simulink model "y005"  (R2019b)
settings: Solver=ode23tb  StartTime=0.0  StopTime=1  MaxStep=0.00001  RelTol=1e-3
values from neighbouring files (symbols this model uses):
  fN = 50    [parameter.m]
  J = 0.1284    [parameter.m]
  Llr = Lr - Lm    (= 0.006)    [parameter.m]
  Lls = Ls - Lm    (= 0.0102)    [parameter.m]
  np = 2    [parameter.m]
  PN = 3000    [parameter.m]
  Rr = 2.685    [parameter.m]
  Rs = 1.85    [parameter.m]
  TN = PN/(2*pi*nN/60)    (= 20.4627783975)    [parameter.m]
  UN = 380    [parameter.m]
undefined symbols (not defined in the file or in its folder): i
libraries: simulink x9, powerlib x9
Description:
  | SVPWM调制
settings Model: Creator=Inspiron  LastModifiedBy=Inspiron
settings SolverCC: ZeroCrossAlgorithm=Adaptive
settings DebuggingCC: IgnoredZcDiagnostic=none

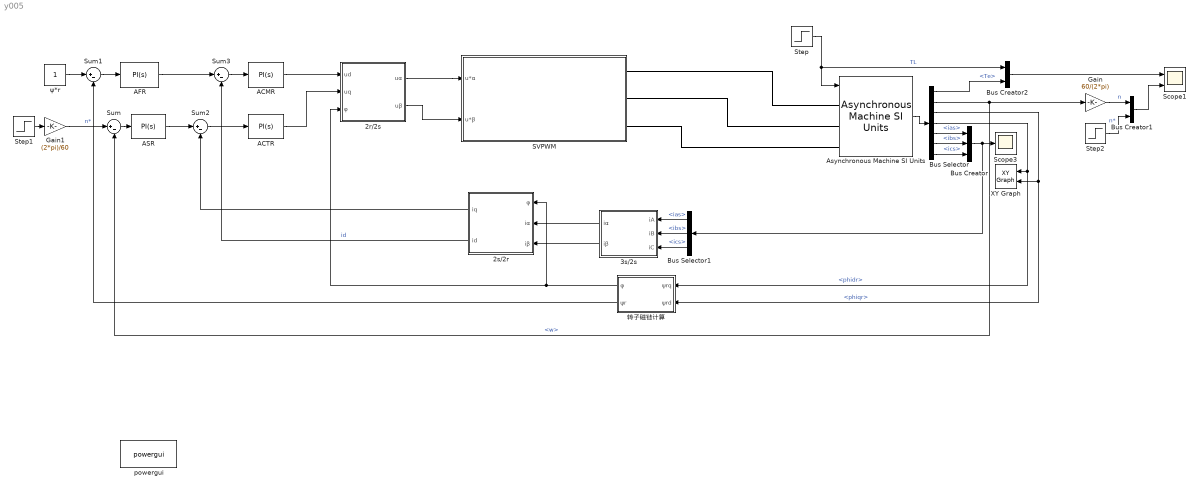
== system y005 ==
  2r/2s : Subsystem
  2s/2r : Subsystem
  3s/2s : Subsystem
  ACMR : simulink/Continuous/PID Controller  Controller=PI  Form=Parallel  TimeDomain=Continuous-time  SampleTime=-1  IntegratorMethod=Forward Euler  FilterMethod=Forward Euler  ControllerParametersSource=internal  P=30  I=2  D=0  UseFilter=on  N=100  TunerSelectOption=Transfer Function Based (PID Tuner App)  InitialConditionSource=internal  InitialConditionForIntegrator=0  InitialConditionForFilter=0  DifferentiatorICPrevScaledInput=0  ExternalReset=none  TrackingMode=off  Kt=1  LimitOutput=on  UpperSaturationLimit=500  LowerSaturationLimit=-500  LinearizeAsGain=on  AntiWindupMode=none  Kb=1  POutMin=[]  POutMax=[]  IOutMin=[]  IOutMax=[]  DOutMin=[]  DOutMax=[]  NOutMin=[]  NOutMax=[]  SumOutMin=[]  SumOutMax=[]  SaturationOutMin=[]  SaturationOutMax=[]  PParamMin=[]  PParamMax=[]  IParamMin=[]  IParamMax=[]  DParamMin=[]  DParamMax=[]  NParamMin=[]  NParamMax=[]  KbParamMin=[]  KbParamMax=[]  KtParamMin=[]  KtParamMax=[]  KbOutMin=[]  KbOutMax=[]  KtOutMin=[]  KtOutMax=[]  IntegratorOutMin=[]  IntegratorOutMax=[]  FilterOutMin=[]  FilterOutMax=[]  SumI1OutMin=[]  SumI1OutMax=[]  SumI2OutMin=[]  SumI2OutMax=[]  SumI3OutMin=[]  SumI3OutMax=[]  SumI4OutMin=[]  SumI4OutMax=[]  SumDOutMin=[]  SumDOutMax=[]  DifferentiatorOutMin=[]  DifferentiatorOutMax=[]  FilterDiffOutCoefMin=[]  FilterDiffOutCoefMax=[]  ReciprocalOutMin=[]  ReciprocalOutMax=[]  SumDenOutMin=[]  SumDenOutMax=[]  SumNumOutMin=[]  SumNumOutMax=[]  DivideOutMin=[]  DivideOutMax=[]  IntegratorContinuousStateAttributes=''  IntegratorStateMustResolveToSignalObject=off  IntegratorRTWStateStorageClass=Auto  FilterContinuousStateAttributes=''  FilterStateMustResolveToSignalObject=off  FilterRTWStateStorageClass=Auto  ParallelPVariant=InternalParameters  IdealPVariant=Disabled  IVariant=InternalParameters  DVariant=Disabled  IntegratorVariant=Continuous  SatVariant=Enabled  AWVariant=Passthrough  PCopyVariant=Disabled  TRVariant=Disabled  FdbkBlocksVariant=Forward  IdealPFdbkVariant=Disabled  SatFdbkVariant=Disabled  DerivativeFilterVariant=Disabled  NVariant=Disabled  NCopyVariant=Disabled_SignalSpec  FilterICVariant=Disabled  IntegratorICVariant=InternalICs  ExternalResetVariant=Disabled  TRSumVariant=Passthrough  SumFdbkVariant=Disabled  SumVariant=Sum_PI
  ACTR : simulink/Continuous/PID Controller  Controller=PI  Form=Parallel  TimeDomain=Continuous-time  SampleTime=-1  IntegratorMethod=Forward Euler  FilterMethod=Forward Euler  ControllerParametersSource=internal  P=50  I=10  D=0  UseFilter=on  N=100  TunerSelectOption=Transfer Function Based (PID Tuner App)  InitialConditionSource=internal  InitialConditionForIntegrator=0  InitialConditionForFilter=0  DifferentiatorICPrevScaledInput=0  ExternalReset=none  TrackingMode=off  Kt=1  LimitOutput=on  UpperSaturationLimit=500  LowerSaturationLimit=-500  LinearizeAsGain=on  AntiWindupMode=none  Kb=1  POutMin=[]  POutMax=[]  IOutMin=[]  IOutMax=[]  DOutMin=[]  DOutMax=[]  NOutMin=[]  NOutMax=[]  SumOutMin=[]  SumOutMax=[]  SaturationOutMin=[]  SaturationOutMax=[]  PParamMin=[]  PParamMax=[]  IParamMin=[]  IParamMax=[]  DParamMin=[]  DParamMax=[]  NParamMin=[]  NParamMax=[]  KbParamMin=[]  KbParamMax=[]  KtParamMin=[]  KtParamMax=[]  KbOutMin=[]  KbOutMax=[]  KtOutMin=[]  KtOutMax=[]  IntegratorOutMin=[]  IntegratorOutMax=[]  FilterOutMin=[]  FilterOutMax=[]  SumI1OutMin=[]  SumI1OutMax=[]  SumI2OutMin=[]  SumI2OutMax=[]  SumI3OutMin=[]  SumI3OutMax=[]  SumI4OutMin=[]  SumI4OutMax=[]  SumDOutMin=[]  SumDOutMax=[]  DifferentiatorOutMin=[]  DifferentiatorOutMax=[]  FilterDiffOutCoefMin=[]  FilterDiffOutCoefMax=[]  ReciprocalOutMin=[]  ReciprocalOutMax=[]  SumDenOutMin=[]  SumDenOutMax=[]  SumNumOutMin=[]  SumNumOutMax=[]  DivideOutMin=[]  DivideOutMax=[]  IntegratorContinuousStateAttributes=''  IntegratorStateMustResolveToSignalObject=off  IntegratorRTWStateStorageClass=Auto  FilterContinuousStateAttributes=''  FilterStateMustResolveToSignalObject=off  FilterRTWStateStorageClass=Auto  ParallelPVariant=InternalParameters  IdealPVariant=Disabled  IVariant=InternalParameters  DVariant=Disabled  IntegratorVariant=Continuous  SatVariant=Enabled  AWVariant=Passthrough  PCopyVariant=Disabled  TRVariant=Disabled  FdbkBlocksVariant=Forward  IdealPFdbkVariant=Disabled  SatFdbkVariant=Disabled  DerivativeFilterVariant=Disabled  NVariant=Disabled  NCopyVariant=Disabled_SignalSpec  FilterICVariant=Disabled  IntegratorICVariant=InternalICs  ExternalResetVariant=Disabled  TRSumVariant=Passthrough  SumFdbkVariant=Disabled  SumVariant=Sum_PI
  AFR : simulink/Continuous/PID Controller  Controller=PI  Form=Parallel  TimeDomain=Continuous-time  SampleTime=-1  IntegratorMethod=Forward Euler  FilterMethod=Forward Euler  ControllerParametersSource=internal  P=80  I=20  D=0  UseFilter=on  N=100  TunerSelectOption=Transfer Function Based (PID Tuner App)  InitialConditionSource=internal  InitialConditionForIntegrator=0  InitialConditionForFilter=0  DifferentiatorICPrevScaledInput=0  ExternalReset=none  TrackingMode=off  Kt=1  LimitOutput=on  UpperSaturationLimit=40  LowerSaturationLimit=-40  LinearizeAsGain=on  AntiWindupMode=none  Kb=1  POutMin=[]  POutMax=[]  IOutMin=[]  IOutMax=[]  DOutMin=[]  DOutMax=[]  NOutMin=[]  NOutMax=[]  SumOutMin=[]  SumOutMax=[]  SaturationOutMin=[]  SaturationOutMax=[]  PParamMin=[]  PParamMax=[]  IParamMin=[]  IParamMax=[]  DParamMin=[]  DParamMax=[]  NParamMin=[]  NParamMax=[]  KbParamMin=[]  KbParamMax=[]  KtParamMin=[]  KtParamMax=[]  KbOutMin=[]  KbOutMax=[]  KtOutMin=[]  KtOutMax=[]  IntegratorOutMin=[]  IntegratorOutMax=[]  FilterOutMin=[]  FilterOutMax=[]  SumI1OutMin=[]  SumI1OutMax=[]  SumI2OutMin=[]  SumI2OutMax=[]  SumI3OutMin=[]  SumI3OutMax=[]  SumI4OutMin=[]  SumI4OutMax=[]  SumDOutMin=[]  SumDOutMax=[]  DifferentiatorOutMin=[]  DifferentiatorOutMax=[]  FilterDiffOutCoefMin=[]  FilterDiffOutCoefMax=[]  ReciprocalOutMin=[]  ReciprocalOutMax=[]  SumDenOutMin=[]  SumDenOutMax=[]  SumNumOutMin=[]  SumNumOutMax=[]  DivideOutMin=[]  DivideOutMax=[]  IntegratorContinuousStateAttributes=''  IntegratorStateMustResolveToSignalObject=off  IntegratorRTWStateStorageClass=Auto  FilterContinuousStateAttributes=''  FilterStateMustResolveToSignalObject=off  FilterRTWStateStorageClass=Auto  ParallelPVariant=InternalParameters  IdealPVariant=Disabled  IVariant=InternalParameters  DVariant=Disabled  IntegratorVariant=Continuous  SatVariant=Enabled  AWVariant=Passthrough  PCopyVariant=Disabled  TRVariant=Disabled  FdbkBlocksVariant=Forward  IdealPFdbkVariant=Disabled  SatFdbkVariant=Disabled  DerivativeFilterVariant=Disabled  NVariant=Disabled  NCopyVariant=Disabled_SignalSpec  FilterICVariant=Disabled  IntegratorICVariant=InternalICs  ExternalResetVariant=Disabled  TRSumVariant=Passthrough  SumFdbkVariant=Disabled  SumVariant=Sum_PI
  ASR : simulink/Continuous/PID Controller  Controller=PI  Form=Parallel  TimeDomain=Continuous-time  SampleTime=-1  IntegratorMethod=Forward Euler  FilterMethod=Forward Euler  ControllerParametersSource=internal  P=15  I=5  D=0  UseFilter=on  N=100  TunerSelectOption=Transfer Function Based (PID Tuner App)  InitialConditionSource=internal  InitialConditionForIntegrator=0  InitialConditionForFilter=0  DifferentiatorICPrevScaledInput=0  ExternalReset=none  TrackingMode=off  Kt=1  LimitOutput=on  UpperSaturationLimit=40  LowerSaturationLimit=-40  LinearizeAsGain=on  AntiWindupMode=none  Kb=1  POutMin=[]  POutMax=[]  IOutMin=[]  IOutMax=[]  DOutMin=[]  DOutMax=[]  NOutMin=[]  NOutMax=[]  SumOutMin=[]  SumOutMax=[]  SaturationOutMin=[]  SaturationOutMax=[]  PParamMin=[]  PParamMax=[]  IParamMin=[]  IParamMax=[]  DParamMin=[]  DParamMax=[]  NParamMin=[]  NParamMax=[]  KbParamMin=[]  KbParamMax=[]  KtParamMin=[]  KtParamMax=[]  KbOutMin=[]  KbOutMax=[]  KtOutMin=[]  KtOutMax=[]  IntegratorOutMin=[]  IntegratorOutMax=[]  FilterOutMin=[]  FilterOutMax=[]  SumI1OutMin=[]  SumI1OutMax=[]  SumI2OutMin=[]  SumI2OutMax=[]  SumI3OutMin=[]  SumI3OutMax=[]  SumI4OutMin=[]  SumI4OutMax=[]  SumDOutMin=[]  SumDOutMax=[]  DifferentiatorOutMin=[]  DifferentiatorOutMax=[]  FilterDiffOutCoefMin=[]  FilterDiffOutCoefMax=[]  ReciprocalOutMin=[]  ReciprocalOutMax=[]  SumDenOutMin=[]  SumDenOutMax=[]  SumNumOutMin=[]  SumNumOutMax=[]  DivideOutMin=[]  DivideOutMax=[]  IntegratorContinuousStateAttributes=''  IntegratorStateMustResolveToSignalObject=off  IntegratorRTWStateStorageClass=Auto  FilterContinuousStateAttributes=''  FilterStateMustResolveToSignalObject=off  FilterRTWStateStorageClass=Auto  ParallelPVariant=InternalParameters  IdealPVariant=Disabled  IVariant=InternalParameters  DVariant=Disabled  IntegratorVariant=Continuous  SatVariant=Enabled  AWVariant=Passthrough  PCopyVariant=Disabled  TRVariant=Disabled  FdbkBlocksVariant=Forward  IdealPFdbkVariant=Disabled  SatFdbkVariant=Disabled  DerivativeFilterVariant=Disabled  NVariant=Disabled  NCopyVariant=Disabled_SignalSpec  FilterICVariant=Disabled  IntegratorICVariant=InternalICs  ExternalResetVariant=Disabled  TRSumVariant=Passthrough  SumFdbkVariant=Disabled  SumVariant=Sum_PI
  Asynchronous Machine SI Units : powerlib/Machines/Asynchronous Machine SI Units  RotorType=Squirrel-cage  PresetModel=No  MechanicalLoad=Torque Tm  ShowDetailedParameters=on  ReferenceFrame=Stationary  Units=SI  MeasurementBus=on  NominalParameters=[PN UN fN]  Stator=[Rs Lls]  Rotor=[Rr Llr]  Cage1=[0.4155 0.002066]  Cage2=[0.4168 0.0003495]  Lm=Lm  Mechanical=[J 0 np]  PolePairs=2  InitialConditions=[1 0 0 0 0 0 0 0]  SimulateSaturation=off  Saturation=[14.03593122, 27.81365428, 53.79336849, 72.68890987, 97.98006896, 148.6815601, 215.7428561, 302.9841135, 428.7778367 ; 230, 322, 414, 460, 506, 552, 598, 644, 690]  LoadFlowParameters=1492000  TsPowergui=0  TsBlock=-1  IterativeModel=Trapezoidal non iterative  IterativeDiscreteModel=Trapezoidal non iterative  Pmec=1.492e+006
      settings: SourceProductName=Simscape Electrical
  Bus Creator : BusCreator  Inputs=3
  Bus Creator1 : BusCreator  Inputs=2
  Bus Creator2 : BusCreator  Inputs=2
  Bus Selector : BusSelector  OutputSignals=Te,w,phiqr,phidr,ias,ibs,ics
  Bus Selector1 : BusSelector  OutputSignals=ias,ibs,ics
  Gain : Gain  Gain=60/(2*pi)
  Gain1 : Gain  Gain=(2*pi)/60
  SVPWM : Subsystem
  Scope1 : Scope  NumInputPorts=2
  Scope3 : Scope
  Step : Step  Time=0.4  After=TN  VectorParams1D=off  ZeroCross=off
  Step1 : Step  Time=0.6  Before=1000  After=0  SampleTime=0
  Step2 : Step  Time=0.6  Before=1000  After=0  SampleTime=0
  Sum{,1..3} (4 alike) : Sum  Inputs=|+-
  XY Graph : simulink/Sinks/XY Graph  xmin=-2  xmax=2  ymin=-2  ymax=2  st=-1
  powergui : powerlib/powergui  Priority=1  SimulationMode=Discrete  SampleTime=1e-5  frequency=60  Iterations=50  frequencyindice=50  Pbase=100e6  ErrMax=1e-4  UnitsV=kV  UnitsW=MW  buscounter=0  FunctionMessages=off  echomessages=off  EnableUseOfTLC=off  CurrentSourceSwitches=off  DisableSnubberDevices=off  DisableRonSwitches=off  DisableVfSwitches=off  DisplayEquations=off  AutomaticDiscreteSolvers=off  SolverType=Tustin/Backward Euler (TBE)  Interpol=off  ExternalGateDelay=off  methode=off  Ts=100  x0status=blocks  SPID=on  SwTol=0  HookPort=off  NonlinearTolerance=1e-4  nMaxIteration=100  ContinueOnMaxIteration=off  RestoreLinks=warning  ResistiveCurrentMeasurement=off  Frange=[0:2:500]  Ylog=off  Xlog=on  ShowGrid=off  save=off  variable=ZData  structure=0  ZoomFFT=off  StartTime=0.0  cycles=1  DisplayStyle=1  fundamental=60  FreqAxis=off  MaxFrequency=1000  frequencyindicesteady=1  RmsSteady=1  display=off
      settings: SourceProductName=Simscape Electrical
  ψ*r : Constant
  转子磁链计算 : Subsystem
  wires:
  Asynchronous Machine SI Units/1 -> Bus Selector/1
  Bus Creator/1 -> Scope3/1, Bus Selector1/1
  Bus Selector/5 -> Bus Creator/1  "<ias>"
  Bus Selector/6 -> Bus Creator/2  "<ibs>"
  Bus Selector/7 -> Bus Creator/3  "<ics>"
  Bus Selector/3 -> 转子磁链计算/2(ψrd), XY Graph/2  "<phiqr>"
  Bus Selector/4 -> 转子磁链计算/1(ψrq), XY Graph/1  "<phidr>"
  Sum/1 -> ASR/1
  ψ*r/1 -> Sum1/1
  Sum1/1 -> AFR/1
  Step/1 -> Bus Creator2/1, Asynchronous Machine SI Units/1  "TL"
  Step2/1 -> Bus Creator1/2  "n*"
  Bus Selector/1 -> Bus Creator2/2  "<Te>"
  Bus Creator2/1 -> Scope1/1
  Bus Creator1/1 -> Scope1/2
  Bus Selector1/1 -> 3s/2s/1(iA)  "<ias>"
  Bus Selector1/3 -> 3s/2s/3(iC)  "<ics>"
  Bus Selector1/2 -> 3s/2s/2(iB)  "<ibs>"
  Gain/1 -> Bus Creator1/1  "n"
  Bus Selector/2 -> Gain/1, Sum/2  "<w>"
  Gain1/1 -> Sum/1  "n*"
  Step1/1 -> Gain1/1
  3s/2s/1(iα) -> 2s/2r/2(iα)
  3s/2s/2(iβ) -> 2s/2r/3(iβ)
  转子磁链计算/1(φ) -> 2s/2r/1(φ), 2r/2s/3(φ)
  转子磁链计算/2(ψr) -> Sum1/2
  ASR/1 -> Sum2/1
  2s/2r/1(iq) -> Sum2/2
  AFR/1 -> Sum3/1
  2s/2r/2(id) -> Sum3/2  "id"
  Sum3/1 -> ACMR/1
  Sum2/1 -> ACTR/1
  ACMR/1 -> 2r/2s/1(ud)
  ACTR/1 -> 2r/2s/2(uq)
  2r/2s/1(uα) -> SVPWM/1(u*α)
  2r/2s/2(uβ) -> SVPWM/2(u*β)
  connections:
  Asynchronous Machine SI Units/LConn1 -- SVPWM/RConn1
  Asynchronous Machine SI Units/LConn2 -- SVPWM/RConn2
  SVPWM/RConn3 -- Asynchronous Machine SI Units/LConn3

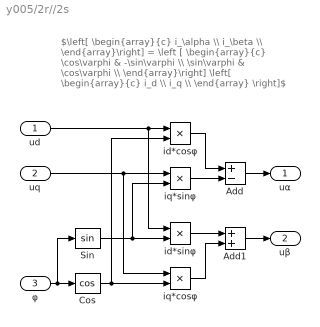
== system y005/2r//2s ==
  note: $\left[ \begin{array}{c} i_\alpha \\ i_\beta \\ \end{array}\right] = \left [ \begin{array}{c} \cos\varphi & -\sin\varphi \\ \sin\varphi & \cos\varphi \\ \end{array}\right] \left[ \begin{array}{c} i_d \\ i_q \\ \end{array} \right]$
  ud : Inport
  uq : Inport  Port=2
  φ : Inport  Port=3
  Add : Sum  Inputs=+-
  Add1 : Sum
  Cos : Trigonometry  Operator=cos
  Sin : Trigonometry
  id*cosφ : Product
  id*sinφ : Product
  iq*cosφ : Product
  iq*sinφ : Product
  uα : Outport
  uβ : Outport  Port=2
  wires:
  Cos/1 -> iq*cosφ/2, id*cosφ/2
  iq*cosφ/1 -> Add1/2
  Sin/1 -> id*sinφ/2, iq*sinφ/2
  ud/1 -> id*cosφ/1, id*sinφ/1
  id*sinφ/1 -> Add1/1
  iq*sinφ/1 -> Add/2
  uq/1 -> iq*sinφ/1, iq*cosφ/1
  φ/1 -> Sin/1, Cos/1
  Add/1 -> uα/1
  id*cosφ/1 -> Add/1
  Add1/1 -> uβ/1

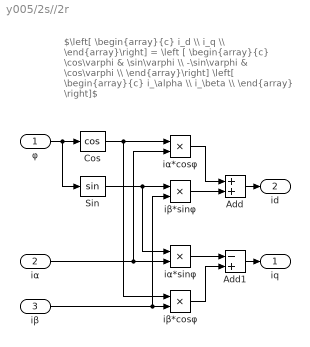
== system y005/2s//2r ==
  note: $\left[ \begin{array}{c} i_d \\ i_q \\ \end{array}\right] = \left [ \begin{array}{c} \cos\varphi & \sin\varphi \\ -\sin\varphi & \cos\varphi \\ \end{array}\right] \left[ \begin{array}{c} i_\alpha \\ i_\beta \\ \end{array} \right]$
  φ : Inport
  iα : Inport  Port=2
  iβ : Inport  Port=3
  Add : Sum
  Add1 : Sum  Inputs=-+
  Cos : Trigonometry  Operator=cos
  Sin : Trigonometry
  iα*cosφ : Product
  iα*sinφ : Product
  iβ*cosφ : Product
  iβ*sinφ : Product
  iq : Outport
  id : Outport  Port=2
  wires:
  Cos/1 -> iα*cosφ/1, iβ*cosφ/1
  iβ*cosφ/1 -> Add1/2
  Sin/1 -> iα*sinφ/1, iβ*sinφ/1
  iα/1 -> iα*sinφ/2, iα*cosφ/2
  iα*sinφ/1 -> Add1/1
  iβ*sinφ/1 -> Add/2
  iβ/1 -> iβ*sinφ/2, iβ*cosφ/2
  φ/1 -> Cos/1, Sin/1
  Add/1 -> id/1
  iα*cosφ/1 -> Add/1
  Add1/1 -> iq/1

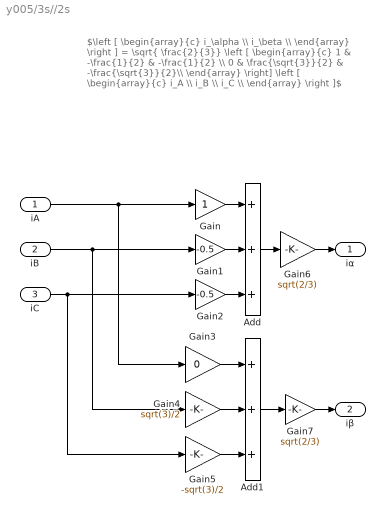
== system y005/3s//2s ==
  note: $\left [ \begin{array}{c} i_\alpha \\ i_\beta \\ \end{array} \right ] = \sqrt{ \frac{2}{3}} \left [ \begin{array}{c} 1 & -\frac{1}{2} & -\frac{1}{2} \\ 0 & \frac{\sqrt{3}}{2} & -\frac{\sqrt{3}}{2}\\ \end{array} \right] \left [ \begin{array}{c} i_A \\ i_B \\ i_C \\ \end{array} \right ]$
  iA : Inport
  iB : Inport  Port=2
  iC : Inport  Port=3
  Add : Sum  Inputs=3
  Add1 : Sum  Inputs=3
  Gain : Gain
  Gain1 : Gain  Gain=-0.5
  Gain2 : Gain  Gain=-0.5
  Gain3 : Gain  Gain=0
  Gain4 : Gain  Gain=sqrt(3)/2
  Gain5 : Gain  Gain=-sqrt(3)/2
  Gain6 : Gain  Gain=sqrt(2/3)
  Gain7 : Gain  Gain=sqrt(2/3)
  iα : Outport
  iβ : Outport  Port=2
  wires:
  Gain4/1 -> Add1/2
  Gain/1 -> Add/1
  Gain5/1 -> Add1/3
  iB/1 -> Gain4/1, Gain1/1
  Add/1 -> Gain6/1
  Gain1/1 -> Add/2
  Gain3/1 -> Add1/1
  iA/1 -> Gain3/1, Gain/1
  Gain2/1 -> Add/3
  iC/1 -> Gain5/1, Gain2/1
  Add1/1 -> Gain7/1
  Gain7/1 -> iβ/1
  Gain6/1 -> iα/1

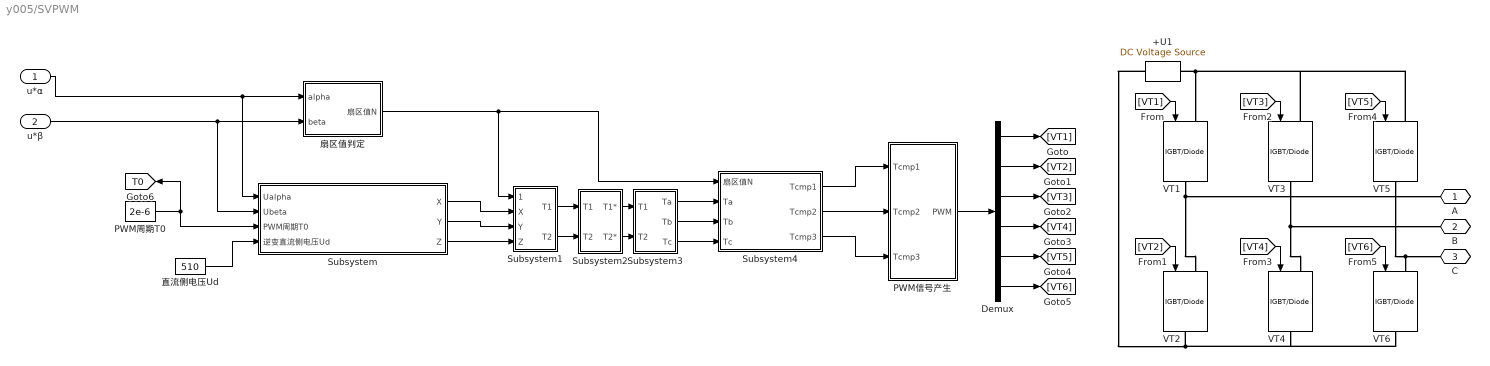
== system y005/SVPWM ==
  u*α : Inport
  u*β : Inport  Port=2
  +U1 : powerlib/Electrical Sources/DC Voltage Source  Amplitude=510  Measurements=None
      settings: SourceProductName=Simscape Electrical
  Demux : Demux  Outputs=6
  PWM信号产生 : Subsystem
  PWM周期T0 : Constant  Value=2e-6
  Subsystem : Subsystem
  Subsystem1 : Subsystem
  Subsystem2 : Subsystem
  Subsystem3 : Subsystem
  Subsystem4 : Subsystem
  VT{1..6} (6 alike) : powerlib/Power Electronics/IGBT//Diode  Ron=1e-3  Rs=1e5  Cs=inf  Measurements=off
      settings: SourceProductName=Simscape Electrical
  扇区值判定 : Subsystem
  直流侧电压Ud : Constant  Value=510
  A : PMIOPort  Side=Right
  B : PMIOPort  Port=2  Side=Right
  C : PMIOPort  Port=3  Side=Right
  tag scope: T0=global
  wires:
  [VT3] -> VT3/1
  [VT4] -> VT4/1
  [VT5] -> VT5/1
  Demux/6 -> [VT6]
  Demux/4 -> [VT4]
  [VT6] -> VT6/1
  [VT2] -> VT2/1
  Demux/2 -> [VT2]
  [VT1] -> VT1/1
  u*β/1 -> 扇区值判定/2(beta), Subsystem/2(Ubeta)
  直流侧电压Ud/1 -> Subsystem/4(逆变直流侧电压Ud)
  u*α/1 -> Subsystem/1(Ualpha), 扇区值判定/1(alpha)
  PWM周期T0/1 -> Subsystem/3(PWM周期T0), [T0]
  Subsystem1/2(T2) -> Subsystem2/2(T2)
  Subsystem4/1(Tcmp1) -> PWM信号产生/1(Tcmp1)
  Subsystem1/1(T1) -> Subsystem2/1(T1)
  Subsystem/2(Y) -> Subsystem1/3(Y)
  Subsystem3/2(Tb) -> Subsystem4/3(Tb)
  Subsystem/3(Z) -> Subsystem1/4(Z)
  Subsystem3/3(Tc) -> Subsystem4/4(Tc)
  Subsystem4/3(Tcmp3) -> PWM信号产生/3(Tcmp3)
  扇区值判定/1(扇区值N) -> Subsystem1/1(扇区值N), Subsystem4/1(扇区值N)
  Subsystem2/2(T2*) -> Subsystem3/2(T2)
  Subsystem3/1(Ta) -> Subsystem4/2(Ta)
  Subsystem/1(X) -> Subsystem1/2(X)
  Subsystem4/2(Tcmp2) -> PWM信号产生/2(Tcmp2)
  Subsystem2/1(T1*) -> Subsystem3/1(T1)
  PWM信号产生/1(PWM) -> Demux/1
  Demux/1 -> [VT1]
  Demux/3 -> [VT3]
  Demux/5 -> [VT5]
  connections:
  +U1/RConn1 -- VT3/LConn1 -- VT5/LConn1 -- VT1/LConn1
  VT6/RConn1 -- VT4/RConn1 -- +U1/LConn1 -- VT2/RConn1
  VT5/RConn1 -- C/RConn1 -- VT6/LConn1
  VT3/RConn1 -- VT4/LConn1 -- B/RConn1
  VT1/RConn1 -- VT2/LConn1 -- A/RConn1

== system y005/转子磁链计算 ==
  ψrq : Inport
  ψrd : Inport  Port=2
  Complex to Magnitude-Angle : ComplexToMagnitudeAngle
  Gain1 : Gain  Gain=-i
  Real-Imag to Complex : RealImagToComplex
  φ : Outport
  ψr : Outport  Port=2
  wires:
  Gain1/1 -> Complex to Magnitude-Angle/1
  Real-Imag to Complex/1 -> Gain1/1
  ψrd/1 -> Real-Imag to Complex/2
  ψrq/1 -> Real-Imag to Complex/1
  Complex to Magnitude-Angle/2 -> φ/1
  Complex to Magnitude-Angle/1 -> ψr/1

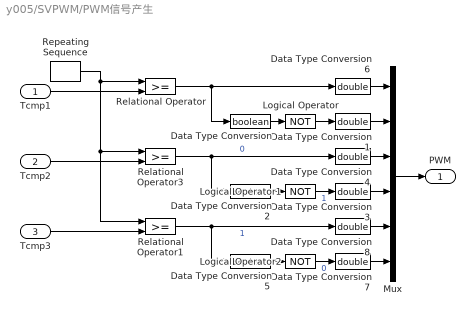
== system y005/SVPWM/PWM信号产生 ==
  Tcmp1 : Inport
  Tcmp2 : Inport  Port=2
  Tcmp3 : Inport  Port=3
  Data Type Conversion : DataTypeConversion  OutDataTypeStr=boolean
  Data Type Conversion{1,3..4,6..8} (6 alike) : DataTypeConversion  OutDataTypeStr=double
  Data Type Conversion2 : DataTypeConversion  OutDataTypeStr=boolean
  Data Type Conversion5 : DataTypeConversion  OutDataTypeStr=boolean
  Logical Operator : Logic  Operator=NOT  AllPortsSameDT=off  OutDataTypeStr=boolean
  Logical Operator1 : Logic  Operator=NOT  AllPortsSameDT=off  OutDataTypeStr=boolean
  Logical Operator2 : Logic  Operator=NOT  AllPortsSameDT=off  OutDataTypeStr=boolean
  Mux : Mux  Inputs=6
  Relational Operator : RelationalOperator  OutDataTypeStr=boolean  RndMeth=Nearest
  Relational Operator1 : RelationalOperator  OutDataTypeStr=boolean  RndMeth=Nearest
  Relational Operator3 : RelationalOperator  OutDataTypeStr=boolean  RndMeth=Nearest
  Repeating Sequence : simulink/Sources/Repeating Sequence  rep_seq_t=[0 1e-4 2e-4]  rep_seq_y=[0 1.3e-6 0]
  PWM : Outport  VectorParamsAs1DForOutWhenUnconnected=off
  wires:
  Data Type Conversion/1 -> Logical Operator/1
  Logical Operator/1 -> Data Type Conversion1/1
  Relational Operator/1 -> Data Type Conversion6/1, Data Type Conversion/1
  Logical Operator1/1 -> Data Type Conversion3/1  "1"
  Relational Operator3/1 -> Data Type Conversion4/1, Data Type Conversion2/1  "0"
  Data Type Conversion2/1 -> Logical Operator1/1
  Relational Operator1/1 -> Data Type Conversion8/1, Data Type Conversion5/1  "1"
  Data Type Conversion5/1 -> Logical Operator2/1
  Logical Operator2/1 -> Data Type Conversion7/1  "0"
  Repeating Sequence/1 -> Relational Operator1/1, Relational Operator3/1, Relational Operator/1
  Tcmp1/1 -> Relational Operator/2
  Tcmp2/1 -> Relational Operator3/2
  Tcmp3/1 -> Relational Operator1/2
  Data Type Conversion6/1 -> Mux/1
  Data Type Conversion1/1 -> Mux/2
  Data Type Conversion4/1 -> Mux/3
  Data Type Conversion3/1 -> Mux/4
  Data Type Conversion8/1 -> Mux/5
  Data Type Conversion7/1 -> Mux/6
  Mux/1 -> PWM/1

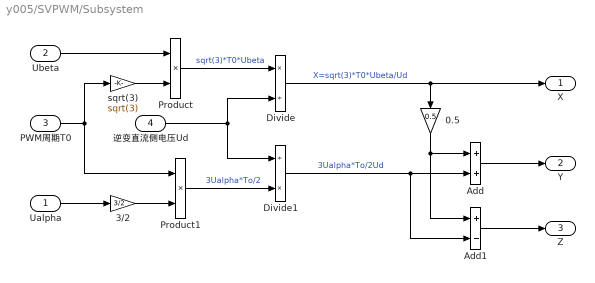
== system y005/SVPWM/Subsystem ==
  Ualpha : Inport
  Ubeta : Inport  Port=2
  PWM周期T0 : Inport  Port=3
  逆变直流侧电压Ud : Inport  Port=4
  0.5 : Gain  Gain=0.5
  3/2 : Gain  Gain=3/2
  Add : Sum
  Add1 : Sum  Inputs=+-
  Divide : Product  Inputs=*/
  Divide1 : Product  Inputs=/*
  Product : Product
  Product1 : Product
  "sqrt(3) " : Gain  Gain=sqrt(3)
  X : Outport  VectorParamsAs1DForOutWhenUnconnected=off
  Y : Outport  Port=2  VectorParamsAs1DForOutWhenUnconnected=off
  Z : Outport  Port=3  VectorParamsAs1DForOutWhenUnconnected=off
  wires:
  Divide/1 -> X/1, 0.5/1  "X=sqrt(3)*T0*Ubeta/Ud"
  逆变直流侧电压Ud/1 -> Divide1/1, Divide/2
  0.5/1 -> Add/1, Add1/1
  PWM周期T0/1 -> "sqrt(3) "/1, Product1/1
  "sqrt(3) "/1 -> Product/2
  3/2/1 -> Product1/2
  Product1/1 -> Divide1/2  "3Ualpha*To/2"
  Add/1 -> Y/1
  Ualpha/1 -> 3/2/1
  Ubeta/1 -> Product/1
  Divide1/1 -> Add1/2, Add/2  "3Ualpha*To/2Ud"
  Add1/1 -> Z/1
  Product/1 -> Divide/1  "sqrt(3)*T0*Ubeta"

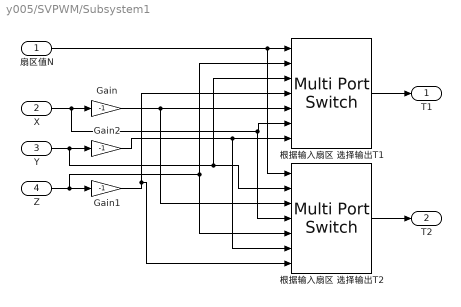
== system y005/SVPWM/Subsystem1 ==
  扇区值N : Inport
  X : Inport  Port=2
  Y : Inport  Port=3
  Z : Inport  Port=4
  Gain : Gain  Gain=-1
  Gain1 : Gain  Gain=-1
  Gain2 : Gain  Gain=-1
  根据输入扇区 选择输出T1 : MultiPortSwitch  Inputs=6
  根据输入扇区 选择输出T2 : MultiPortSwitch  Inputs=6
  T1 : Outport  VectorParamsAs1DForOutWhenUnconnected=off
  T2 : Outport  Port=2  VectorParamsAs1DForOutWhenUnconnected=off
  wires:
  X/1 -> 根据输入扇区 选择输出T2/4, 根据输入扇区 选择输出T1/6, Gain/1
  Y/1 -> 根据输入扇区 选择输出T1/3, 根据输入扇区 选择输出T2/2, Gain2/1
  Z/1 -> 根据输入扇区 选择输出T2/5, 根据输入扇区 选择输出T1/2, Gain1/1
  Gain1/1 -> 根据输入扇区 选择输出T2/7, 根据输入扇区 选择输出T1/4
  Gain/1 -> 根据输入扇区 选择输出T1/5, 根据输入扇区 选择输出T2/3
  根据输入扇区 选择输出T1/1 -> T1/1
  根据输入扇区 选择输出T2/1 -> T2/1
  Gain2/1 -> 根据输入扇区 选择输出T2/6, 根据输入扇区 选择输出T1/7
  扇区值N/1 -> 根据输入扇区 选择输出T2/1, 根据输入扇区 选择输出T1/1

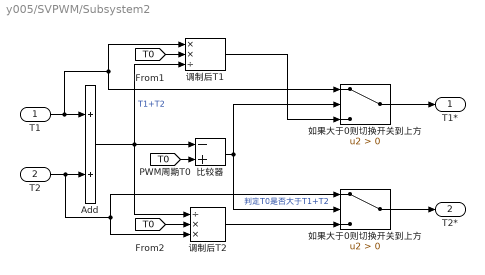
== system y005/SVPWM/Subsystem2 ==
  T1 : Inport
  T2 : Inport  Port=2
  Add : Sum
  如果大于0则切换开关到上方 : Switch  Criteria=u2 > Threshold
  "如果大于0则切换开关到上方 " : Switch  Criteria=u2 > Threshold
  比较器 : Sum  Inputs=-+
  调制后T1 : Product  Inputs=**/
  调制后T2 : Product  Inputs=/**
  T1* : Outport  VectorParamsAs1DForOutWhenUnconnected=off
  T2* : Outport  Port=2  VectorParamsAs1DForOutWhenUnconnected=off
  wires:
  调制后T1/1 -> 如果大于0则切换开关到上方/3
  "如果大于0则切换开关到上方 "/1 -> T2*/1
  比较器/1 -> "如果大于0则切换开关到上方 "/2, 如果大于0则切换开关到上方/2  "判定T0是否大于T1+T2"
  [T0] -> 调制后T2/2
  Add/1 -> 调制后T2/1, 比较器/1, 调制后T1/3  "T1+T2"
  [T0] -> 调制后T1/2
  T1/1 -> 如果大于0则切换开关到上方/1, 调制后T1/1, Add/1
  [T0] -> 比较器/2
  如果大于0则切换开关到上方/1 -> T1*/1
  调制后T2/1 -> "如果大于0则切换开关到上方 "/3
  T2/1 -> "如果大于0则切换开关到上方 "/1, 调制后T2/3, Add/2

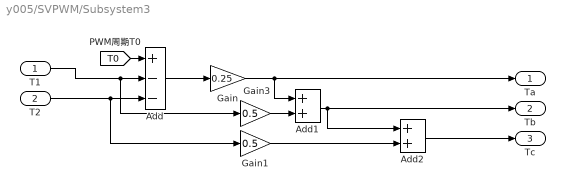
== system y005/SVPWM/Subsystem3 ==
  T1 : Inport
  T2 : Inport  Port=2
  Add : Sum  Inputs=+--
  Add1 : Sum
  Add2 : Sum
  Gain : Gain  Gain=0.25
  Gain1 : Gain  Gain=0.5
  Gain3 : Gain  Gain=0.5
  Ta : Outport  VectorParamsAs1DForOutWhenUnconnected=off
  Tb : Outport  Port=2  VectorParamsAs1DForOutWhenUnconnected=off
  Tc : Outport  Port=3  VectorParamsAs1DForOutWhenUnconnected=off
  wires:
  Add2/1 -> Tc/1
  Add/1 -> Gain/1
  [T0] -> Add/1
  T1/1 -> Gain3/1, Add/2
  Add1/1 -> Tb/1, Add2/1
  Gain3/1 -> Add1/2
  Gain1/1 -> Add2/2
  Gain/1 -> Ta/1, Add1/1
  T2/1 -> Gain1/1, Add/3

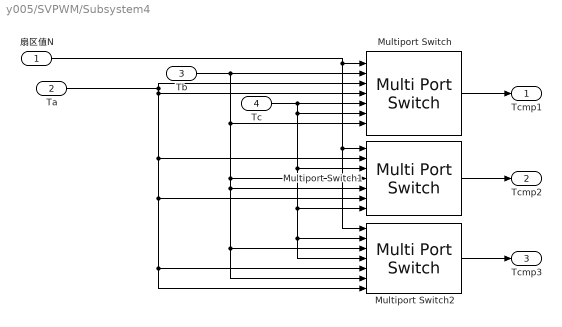
== system y005/SVPWM/Subsystem4 ==
  扇区值N : Inport
  Ta : Inport  Port=2
  Tb : Inport  Port=3
  Tc : Inport  Port=4
  Multiport Switch : MultiPortSwitch  Inputs=6  OutDataTypeStr=double
  Multiport Switch1 : MultiPortSwitch  Inputs=6  OutDataTypeStr=double
  Multiport Switch2 : MultiPortSwitch  Inputs=6  OutDataTypeStr=double
  Tcmp1 : Outport  VectorParamsAs1DForOutWhenUnconnected=off
  Tcmp2 : Outport  Port=2  VectorParamsAs1DForOutWhenUnconnected=off
  Tcmp3 : Outport  Port=3  VectorParamsAs1DForOutWhenUnconnected=off
  wires:
  扇区值N/1 -> Multiport Switch2/1, Multiport Switch1/1, Multiport Switch/1
  Tb/1 -> Multiport Switch2/6, Multiport Switch2/3, Multiport Switch1/5, Multiport Switch1/4, Multiport Switch/7, Multiport Switch/2
  Multiport Switch/1 -> Tcmp1/1
  Ta/1 -> Multiport Switch/3, Multiport Switch/4, Multiport Switch2/7, Multiport Switch2/5, Multiport Switch1/6, Multiport Switch1/2
  Multiport Switch1/1 -> Tcmp2/1
  Tc/1 -> Multiport Switch1/7, Multiport Switch2/2, Multiport Switch2/4, Multiport Switch1/3, Multiport Switch/6, Multiport Switch/5
  Multiport Switch2/1 -> Tcmp3/1

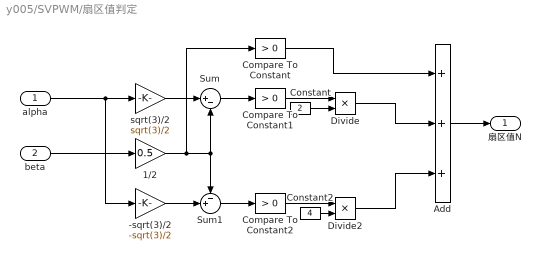
== system y005/SVPWM/扇区值判定 ==
  alpha : Inport
  beta : Inport  Port=2
  -sqrt(3)/2 : Gain  Gain=-sqrt(3)/2
  1/2 : Gain  Gain=0.5
  "Add " : Sum  Inputs=+++
  Compare To Constant : simulink/Logic and Bit Operations/Compare To Constant  relop=>  const=0  OutDataTypeStr=boolean
  Compare To Constant1 : simulink/Logic and Bit Operations/Compare To Constant  relop=>  const=0  OutDataTypeStr=boolean
  Compare To Constant2 : simulink/Logic and Bit Operations/Compare To Constant  relop=>  const=0  OutDataTypeStr=boolean
  Constant : Constant  Value=2
  Constant2 : Constant  Value=4
  Divide : Product  Inputs=**
  Divide2 : Product  Inputs=**
  Sum : Sum  Inputs=|+-
  Sum1 : Sum  Inputs=-+|
  sqrt(3)/2 : Gain  Gain=sqrt(3)/2
  扇区值N : Outport  VectorParamsAs1DForOutWhenUnconnected=off
  wires:
  Divide2/1 -> "Add "/3
  Sum/1 -> Compare To Constant1/1
  -sqrt(3)/2/1 -> Sum1/2
  Sum1/1 -> Compare To Constant2/1
  Constant2/1 -> Divide2/2
  1/2/1 -> Sum1/1, Sum/2, Compare To Constant/1
  "Add "/1 -> 扇区值N/1
  Compare To Constant2/1 -> Divide2/1
  beta/1 -> 1/2/1
  sqrt(3)/2/1 -> Sum/1
  Compare To Constant/1 -> "Add "/1
  Compare To Constant1/1 -> Divide/1
  Divide/1 -> "Add "/2
  Constant/1 -> Divide/2
  alpha/1 -> -sqrt(3)/2/1, sqrt(3)/2/1
